simulink model "Prob01"  (R2020a)
settings: Solver=VariableStepAuto  StartTime=0.0  StopTime=10.0  RelTol=1e-3
model workspace (MAT data in the model file):
  M1 = Simulink.Parameter
  M1.Value = 100
  M1.DataType = 'auto'
  M1.Dimensions = [1 1]
  M2 = Simulink.Parameter
  M2.Value = 0.5
  M2.DataType = 'auto'
  M2.Dimensions = [1 1]
  b = Simulink.Parameter
  b.Value = 50
  b.DataType = 'auto'
  b.Dimensions = [1 1]
  k1 = Simulink.Parameter
  k1.Value = 50
  k1.DataType = 'auto'
  k1.Dimensions = [1 1]
  t = Simulink.Parameter
  t.Value = 10
  t.DataType = 'auto'
  t.Dimensions = [1 1]
settings Model: OrderedModelArguments=off  Creator=Shivam  LastModifiedBy=Shivam

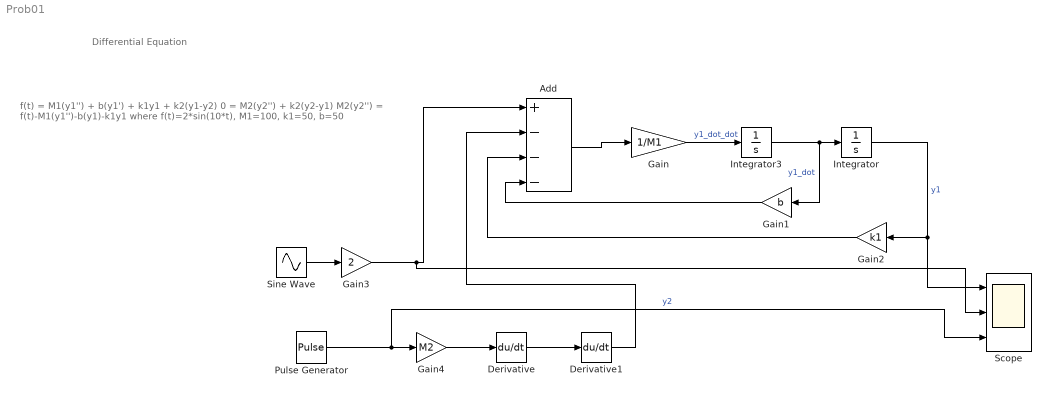
== system Prob01 ==
  note: f(t) = M1(y1'') + b(y1') + k1y1 + k2(y1-y2)
      | 0 = M2(y2'') + k2(y2-y1)
      | M2(y2'') = f(t)-M1(y1'')-b(y1)-k1y1
      | where f(t)=2*sin(10*t), M1=100, k1=50, b=50
  note: Differential Equation
  Add : Sum  Inputs=+---
  Derivative : Derivative
  Derivative1 : Derivative
  Gain : Gain  Gain=1/M1
  Gain1 : Gain  Gain=b
  Gain2 : Gain  Gain=k1
  Gain3 : Gain  Gain=2
  Gain4 : Gain  Gain=M2
  Integrator : Integrator
  Integrator3 : Integrator
  Pulse Generator : DiscretePulseGenerator  PulseType=Time based  Period=10  PulseWidth=5
  Scope : Scope  NumInputPorts=3
  Sine Wave : Sin  Frequency=10*t  SampleTime=0
  wires:
  Integrator3/1 -> Gain1/1, Integrator/1  "y1_dot"
  Integrator/1 -> Scope/1, Gain2/1  "y1"
  Sine Wave/1 -> Gain3/1
  Gain3/1 -> Scope/2, Add/1
  Gain/1 -> Integrator3/1  "y1_dot_dot"
  Gain1/1 -> Add/4
  Gain2/1 -> Add/3
  Add/1 -> Gain/1
  Pulse Generator/1 -> Scope/3, Gain4/1  "y2"
  Gain4/1 -> Derivative/1
  Derivative/1 -> Derivative1/1
  Derivative1/1 -> Add/2
